simulink model "vertical_controller"  (R2020a)
settings: Solver=ode4  StartTime=0.0  StopTime=simtime  FixedStep=0.001  RelTol=1e-3
values from neighbouring files (symbols this model uses):
  desired_energy = M1*g*(H+r1) + M2*g*(H+k0+r2)    (= 185.22)    [fast_vertical_controller.m]
  g = 9.8    [fast_vertical_controller.m]
  H = 0.4    [fast_vertical_controller.m]
  ini_y1 = ini_y0+r1*cos(ini_theta1)    [fast_vertical_controller.m]
  ini_y1_d = 0    [fast_vertical_controller.m]
  ini_y2 = ini_y0+ini_w+r2*cos(ini_theta2)    [fast_vertical_controller.m]
  ini_y2_d = 0    [fast_vertical_controller.m]
  M1 = 1    [fast_vertical_controller.m]
  M2 = 10    [fast_vertical_controller.m]
  r1 = 0.5    [fast_vertical_controller.m]
  r2 = 0.4    [fast_vertical_controller.m]
settings Model: Creator=fabia  LastModifiedBy=mic-ciciolla

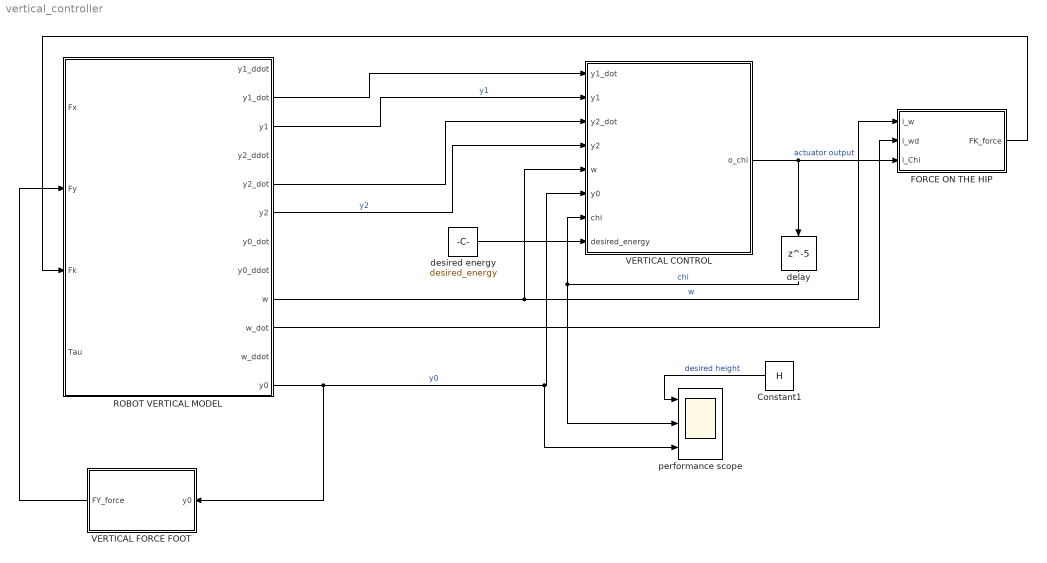
== system vertical_controller ==
  " ROBOT VERTICAL MODEL " : Subsystem
  " VERTICAL FORCE FOOT" : MATLAB Function  TreatAsAtomicUnit=on
  Constant1 : Constant  Value=H
  FORCE ON THE HIP : MATLAB Function  TreatAsAtomicUnit=on
  VERTICAL CONTROL : MATLAB Function  TreatAsAtomicUnit=on
  delay : Delay  DelayLength=5  InitialCondition=0
  desired energy : Constant  Value=desired_energy
  performance scope : Scope  NumInputPorts=3
  wires:
  " VERTICAL FORCE FOOT"/1(FY_force) -> " ROBOT VERTICAL MODEL "/2(Fy)
  FORCE ON THE HIP/1(FK_force) -> " ROBOT VERTICAL MODEL "/3(Fk)
  " ROBOT VERTICAL MODEL "/3(y1) -> VERTICAL CONTROL/2(y1)  "y1"
  " ROBOT VERTICAL MODEL "/2(y1_dot) -> VERTICAL CONTROL/1(y1_dot)
  " ROBOT VERTICAL MODEL "/6(y2) -> VERTICAL CONTROL/4(y2)  "y2"
  " ROBOT VERTICAL MODEL "/5(y2_dot) -> VERTICAL CONTROL/3(y2_dot)
  " ROBOT VERTICAL MODEL "/9(w) -> FORCE ON THE HIP/1(i_w), VERTICAL CONTROL/5(w)  "w"
  " ROBOT VERTICAL MODEL "/10(w_dot) -> FORCE ON THE HIP/2(i_wd)
  delay/1 -> performance scope/2, VERTICAL CONTROL/7(chi)  "chi"
  desired energy/1 -> VERTICAL CONTROL/8(desired_energy)
  " ROBOT VERTICAL MODEL "/12(y0) -> " VERTICAL FORCE FOOT"/1(y0), performance scope/3, VERTICAL CONTROL/6(y0)  "y0"
  VERTICAL CONTROL/1(o_chi) -> FORCE ON THE HIP/3(i_Chi), delay/1  "actuator output"
  Constant1/1 -> performance scope/1  "desired height"

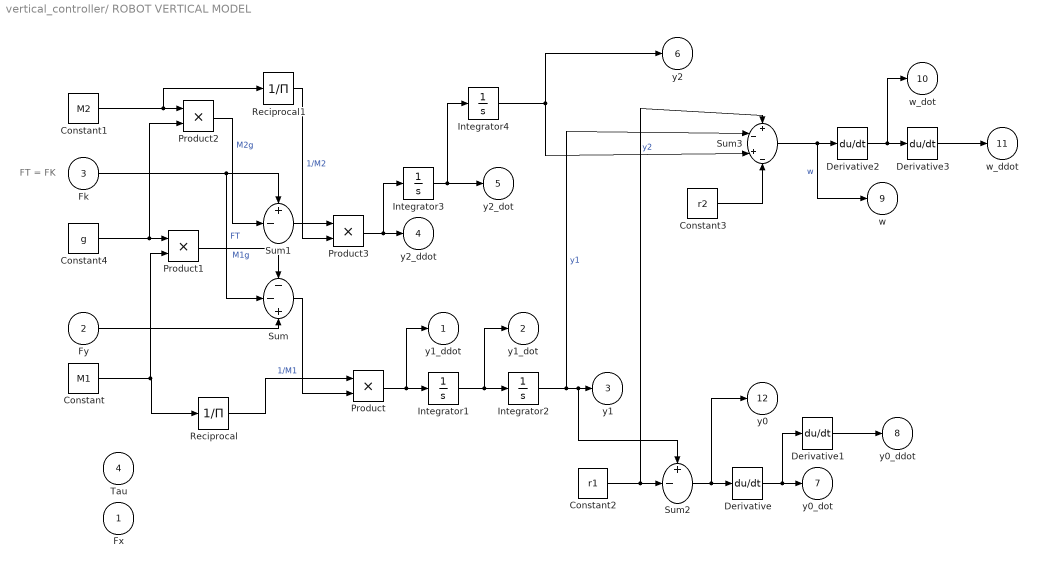
== system vertical_controller/ ROBOT VERTICAL MODEL  ==
  note: FT = FK
  Fx : Inport
  Fy : Inport  Port=2
  Fk : Inport  Port=3
  Tau : Inport  Port=4
  Constant : Constant  Value=M1
  Constant1 : Constant  Value=M2
  Constant2 : Constant  Value=r1
  Constant3 : Constant  Value=r2
  Constant4 : Constant  Value=g
  Derivative{,1..3} (4 alike) : Derivative
  Integrator1 : Integrator  InitialCondition=ini_y1_d
  Integrator2 : Integrator  InitialCondition=ini_y1
  Integrator3 : Integrator  InitialCondition=ini_y2_d
  Integrator4 : Integrator  InitialCondition=ini_y2
  Product{,1..3} (4 alike) : Product
  Reciprocal : Product  Inputs=/
  Reciprocal1 : Product  Inputs=/
  Sum : Sum  Inputs=--+
  Sum1 : Sum  Inputs=+-|
  Sum2 : Sum  Inputs=+-|
  Sum3 : Sum  Inputs=+-+-
  y1_ddot : Outport
  y1_dot : Outport  Port=2
  y1 : Outport  Port=3
  y2_ddot : Outport  Port=4
  y2_dot : Outport  Port=5
  y2 : Outport  Port=6
  y0_dot : Outport  Port=7
  y0_ddot : Outport  Port=8
  w : Outport  Port=9
  w_dot : Outport  Port=10
  w_ddot : Outport  Port=11
  y0 : Outport  Port=12
  wires:
  Constant4/1 -> Product1/1, Product2/2
  Fk/1 -> Sum1/1, Sum/2  "FT"
  Product1/1 -> Sum/1  "M1g"
  Sum/1 -> Product/2
  Reciprocal1/1 -> Product3/2  "1/M2"
  Derivative1/1 -> y0_ddot/1
  Fy/1 -> Sum/3
  Product2/1 -> Sum1/2  "M2g"
  Product/1 -> Integrator1/1, y1_ddot/1
  Integrator4/1 -> y2/1, Sum3/3  "y2"
  Integrator3/1 -> y2_dot/1, Integrator4/1
  Derivative3/1 -> w_ddot/1
  Constant3/1 -> Sum3/4
  Constant2/1 -> Sum2/2, Sum3/1
  Sum1/1 -> Product3/1
  Reciprocal/1 -> Product/1  "1/M1"
  Integrator2/1 -> Sum2/1, y1/1, Sum3/2  "y1"
  Constant/1 -> Reciprocal/1, Product1/2
  Constant1/1 -> Reciprocal1/1, Product2/1
  Sum2/1 -> y0/1, Derivative/1
  Derivative/1 -> Derivative1/1, y0_dot/1
  Integrator1/1 -> Integrator2/1, y1_dot/1
  Derivative2/1 -> Derivative3/1, w_dot/1
  Product3/1 -> Integrator3/1, y2_ddot/1
  Sum3/1 -> w/1, Derivative2/1  "w"

== matlab function vertical_controller/ VERTICAL FORCE FOOT ==
  data: y0 input; FY_force output
function FY_force = Fy(y0)

KG=10^4; % [Nt/m]
BG=75; % [Nt-s/m]

FY_force = 0;

if y0<0 
    FY_force = -KG*y0-BG*y0;
end

== matlab function vertical_controller/VERTICAL CONTROL ==
  data: y1_dot input; y1 input; y2_dot input; y2 input; w input; y0 input; chi input; desired_energy input; o_chi output
function o_chi = Vertical_control(y1_dot,y1,y2_dot,y2,w,y0,chi,desired_energy)

chi_min=0.0;
chi_max=0.15;


M1=1; % Leg mass [kg]
M2=10; % Body mass [kg]

k0=1; % [m]
KL=10^3; % [Nt/m]

KG=10^4; % [Nt/m]
g=9.8;

E_flight=(M2/(M1+M2))*...
    (M1*g*y1+...
    M2*g*y2+...
    0.5*M1*y1_dot^2+...
    0.5*M2*y2_dot^2+...
    0.5*(KL*(k0-w+chi)^2)+...
    0.5*KG*y0^2);

Delta_EH=desired_energy-E_flight;

Delta_chi=-(chi-w+k0)+sqrt((chi-w+k0)^2+((2*abs(Delta_EH))/KL));

if Delta_EH >= 0
    o_chi=chi+Delta_chi;
else
    o_chi=chi-Delta_chi;
end

if o_chi<chi_min
    o_chi=chi_min;
end
if o_chi>chi_max
    o_chi=chi_max;
end





end

== matlab function vertical_controller/FORCE ON THE HIP ==
  data: i_w input; FK_force output; i_wd input; i_Chi input
function FK_force  = FK(i_w,i_wd,i_Chi)

k0=1; % [m]
KL=10^3; % [Nt/m]

KL2=10^5; % [Nt/m]
BL2=125; % [Nt-s/m]

condition = (k0-i_w+i_Chi);

FK_force=KL2*condition-(BL2*i_wd);


if condition>0
    FK_force = KL*condition;
end

    
end
